simulink model "rover"  (R2020b)
settings: Solver=VariableStepAuto  StartTime=0.0  StopTime=10.0  RelTol=1e-3
libraries: pid_lib x1
settings Model: Creator=giuse  LastModifiedBy=giuse

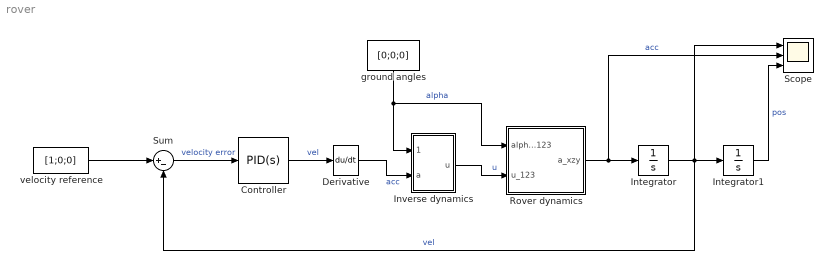
== system rover ==
  Controller : pid_lib/PID Controller  Controller=PID  Form=Parallel  TimeDomain=Continuous-time  UseExternalTs=off  SampleTime=-1  IntegratorMethod=Forward Euler  FilterMethod=Forward Euler  ControllerParametersSource=internal  P=1  I=1  D=0  UseFilter=on  N=100  TunerSelectOption=Transfer Function Based (PID Tuner App)  InitialConditionSource=internal  InitialConditionForIntegrator=0  InitialConditionForFilter=0  DifferentiatorICPrevScaledInput=0  ExternalReset=none  TrackingMode=off  Kt=1  LimitOutput=off  SatLimitsSource=internal  UpperSaturationLimit=inf  LowerSaturationLimit=-inf  LinearizeAsGain=on  AntiWindupMode=none  Kb=1  POutMin=[]  POutMax=[]  IOutMin=[]  IOutMax=[]  DOutMin=[]  DOutMax=[]  NOutMin=[]  NOutMax=[]  SumOutMin=[]  SumOutMax=[]  SaturationOutMin=[]  SaturationOutMax=[]  PParamMin=[]  PParamMax=[]  IParamMin=[]  IParamMax=[]  DParamMin=[]  DParamMax=[]  NParamMin=[]  NParamMax=[]  KbParamMin=[]  KbParamMax=[]  KtParamMin=[]  KtParamMax=[]  KbOutMin=[]  KbOutMax=[]  KtOutMin=[]  KtOutMax=[]  IntegratorOutMin=[]  IntegratorOutMax=[]  FilterOutMin=[]  FilterOutMax=[]  SumI1OutMin=[]  SumI1OutMax=[]  SumI2OutMin=[]  SumI2OutMax=[]  SumI3OutMin=[]  SumI3OutMax=[]  SumI4OutMin=[]  SumI4OutMax=[]  SumDOutMin=[]  SumDOutMax=[]  DifferentiatorOutMin=[]  DifferentiatorOutMax=[]  FilterDiffOutCoefMin=[]  FilterDiffOutCoefMax=[]  ReciprocalOutMin=[]  ReciprocalOutMax=[]  SumDenOutMin=[]  SumDenOutMax=[]  SumNumOutMin=[]  SumNumOutMax=[]  DivideOutMin=[]  DivideOutMax=[]  UdiffTsProdOutMin=[]  UdiffTsProdOutMax=[]  NTsProdOutMin=[]  NTsProdOutMax=[]  UintegralTsProdOutMin=[]  UintegralTsProdOutMax=[]  UngainTsProdOutMin=[]  UngainTsProdOutMax=[]  IntegratorContinuousStateAttributes=''  IntegratorStateMustResolveToSignalObject=off  IntegratorRTWStateStorageClass=Auto  FilterContinuousStateAttributes=''  FilterStateMustResolveToSignalObject=off  FilterRTWStateStorageClass=Auto  ParallelPVariant=InternalParameters  IdealPVariant=Disabled  IVariant=InternalParameters  DVariant=InternalParameters  IntegratorVariant=Continuous  SatVariant=Disabled  AWVariant=Passthrough  PCopyVariant=Disabled  TRVariant=Disabled  FdbkBlocksVariant=Forward  IdealPFdbkVariant=Disabled  SatFdbkVariant=Disabled  DerivativeFilterVariant=ContFilter  NVariant=InternalParameters  NCopyVariant=Disabled  FilterICVariant=InternalICsFilter  IntegratorICVariant=InternalICs  ExternalResetVariant=Disabled  TRSumVariant=Passthrough  SumFdbkVariant=Disabled  SumVariant=Sum_PID  TsampFilterVariant=InternalTs  TsampNgainVariant=Passthrough  TsampIntegralVariant=Passthrough  ExternalSaturationOutDataTypeStr=Inherit: Same as second input
  Derivative : Derivative
  Integrator : Integrator
  Integrator1 : Integrator
  Inverse dynamics : MATLAB Function  TreatAsAtomicUnit=on
  Rover dynamics : Subsystem
  Scope : Scope  NumInputPorts=3
  Sum : Sum  Inputs=|+-
  ground angles : Constant  Value=[0;0;0]
  velocity reference : Constant  Value=[1;0;0]
  wires:
  Sum/1 -> Controller/1  "velocity error"
  Controller/1 -> Derivative/1  "vel"
  Derivative/1 -> Inverse dynamics/2(a)  "acc"
  ground angles/1 -> Rover dynamics/1(alpha_123), Inverse dynamics/1(alpha)  "alpha"
  Inverse dynamics/1(u) -> Rover dynamics/2(u_123)  "u"
  Rover dynamics/1(a_xzy) -> Scope/2, Integrator/1  "acc"
  Integrator/1 -> Integrator1/1, Scope/1, Sum/2  "vel"
  velocity reference/1 -> Sum/1
  Integrator1/1 -> Scope/3  "pos"

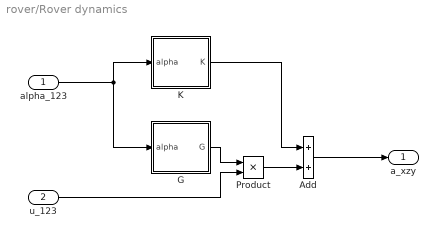
== system rover/Rover dynamics ==
  alpha_123 : Inport
  u_123 : Inport  Port=2
  Add : Sum
  G : MATLAB Function  TreatAsAtomicUnit=on
  K : MATLAB Function  TreatAsAtomicUnit=on
  Product : Product
  a_xzy : Outport
  wires:
  alpha_123/1 -> G/1(alpha), K/1(alpha)
  u_123/1 -> Product/2
  G/1(G) -> Product/1
  K/1(K) -> Add/1
  Add/1 -> a_xzy/1
  Product/1 -> Add/2

== matlab function rover/Inverse dynamics ==
  data: alpha input; u output; a input
function u = fcn(alpha, a)

K = [0;0;0];    % normal forces

u = [-(Im*(ax*cos(alpha1) + az*cos(alpha2) + dwy*cos(alpha3) - K(1)*cos(alpha1) - K(2)*cos(alpha2) - K(3)*cos(alpha3)))/(m*r);
	(Im*(ax*sin(alpha1) + az*sin(alpha2) + dwy*sin(alpha3) - K(1)*sin(alpha1) - K(2)*sin(alpha2) - K(3)*sin(alpha3)))/(m*r);
    -(Im*gamma1*(ax - k1))/(Iy*r)];

== matlab function rover/Rover dynamics/K ==
  data: alpha input; K output
function K = fcn(alpha)

K = [0,0,0];

== matlab function rover/Rover dynamics/G ==
  data: alpha input; G output
function G = fcn(alpha)
G = [0, 0, 0;
    -1/m*((Im/r)*cos(alpha(1))), -1/m*((Im/r)*cos(alpha(2))), -1/m*((Im/r)*cos(alpha(3)));
    0, 0, 0;
    1/m*((Im/r)*sin(alpha(1))), 1/m*((Im/r)*sin(alpha(2))), 1/m*((Im/r)*sin(alpha(3)));
    0, 0, 0;
    -1/Iy*((Im/r)*1), 0, 0]; % gamma1 should be here
